simulink library "commsynccomp2"  (Simulink 6.0)
settings: Solver=ode45  SolverMode=SingleTasking  StartTime=0.0  StopTime=10.0  RelTol=1e-3
libraries: commblksprivate x15, dspsigattribs x10, simulink_extras x2, commcontsrc2 x2, dspsrcs4 x1
settings Model: Creator=akansal  LastModifiedBy=cvora  ExtModeAutoUpdateStatusClock=off
settings DataIOCC: SignalLoggingName=logsOut
settings OptimizationCC: BooleanDataType=off
settings DebuggingCC: CheckExecutionContextPreStartOutputMsg=on  CheckExecutionContextRuntimeOutputMsg=on  SolverPrmCheckMsg=none
settings HardwareCC: TargetUnknown=on
settings SFSimCC: SFSimApplyToAllLibs=on  SFSimBuildMode=Incremental

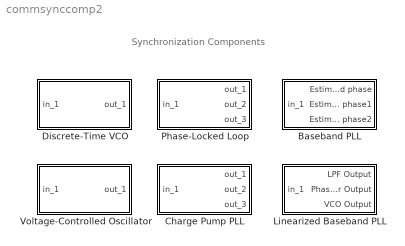
== system commsynccomp2 ==
  note: Synchronization Components
  Baseband PLL : Subsystem  PropExecContextAcrossSSBoundary=on  mask(Baseband PLL){Fn=[3.0002  0  40002], Fd=[1   67.46   2270.9   40002], Kvco=1}
      mask prompts: Fn "Lowpass filter numerator:"; Fd "Lowpass filter denominator:"; Kvco "VCO input sensitivity (Hz/V):"
      mask help: Implement a baseband model of a phase-locked loop. The three outputs are the outputs of the lowpass filter, the phase detector, and the voltage controlled oscillator (VCO). The input must be a sample-based scalar signal.
      mask init:
      | pi2=2*pi;
      mask Help: helpview(commbhelp)
      mask Display:
      | disp('Baseband\nPLL')
      | port_label('output',1,'Filt');
      | port_label('output',2,'PD');
      | port_label('output',3,'VCO');
  Charge Pump PLL : Subsystem  PropExecContextAcrossSSBoundary=on  mask(Charge Pump PLL){Fn=[3.0002  0  40002], Fd=[1   67.46   2270.9   40002], Kvco=1, Fc=100, Ph=0, Ac=1}
      mask prompts: Fn "Lowpass filter numerator:"; Fd "Lowpass filter denominator:"; Kvco "VCO input sensitivity (Hz/V):"; Fc "VCO quiescent frequency (Hz):"; Ph "VCO initial phase (rad):"; Ac "VCO output amplitude (V):"
      mask help: Implement a charge pump phase-locked loop using a digital phase detector. The three outputs are the outputs of the lowpass filter, the phase detector, and the voltage controlled oscillator (VCO). The input must be a sample-based scalar signal.
      mask init:
      | Cu=1;
      mask Help: helpview(commbhelp)
      mask Display:
      | disp('Charge\nPump\nPLL')
      | port_label('output',1,'Filt');
      | port_label('output',2,'PD');
      | port_label('output',3,'VCO');
  Discrete-Time VCO : Subsystem  PropExecContextAcrossSSBoundary=on  mask(Discrete-Time VCO){Ac=1, Fc=10, Kc=1, Ph=0, ts=.01}
      mask prompts: Ac "Output amplitude (V):"; Fc "Quiescent frequency (Hz):"; Kc "Input sensitivity (Hz/V):"; Ph "Initial phase (rad):"; ts "Sample time (s):"
      mask help: Generate a discrete-time output signal whose frequency changes in response to the amplitude variations of the input signal. The input signal must be a scalar.
      mask init:
      | if ((length(Ac)~=1) | (length(Fc)~=1) | (length(Kc)~=1) | (length(Ph)~=1) | (length(ts)~=1))error('Mask parameters must be scalar values.');end;
      | pi2=2*pi;Kc=Kc*pi2*ts(1);Fc=Fc*pi2;
      mask Help: helpview(commbhelp)
      mask Display: disp('Discrete-Time\nVCO')
  Linearized Baseband PLL : Subsystem  PropExecContextAcrossSSBoundary=on  mask(Linearized Baseband PLL){Fn=[3.0002  0  40002], Fd=[1   67.46   2270.9   40002], Kvco=1}
      mask prompts: Fn "Lowpass filter numerator:"; Fd "Lowpass filter denominator:"; Kvco "VCO input sensitivity (Hz/V):"
      mask help: Implement a linearized baseband model of a phase-locked loop. The three outputs are the outputs of the lowpass filter, the phase detector, and the voltage controlled oscillator (VCO). The input must be a sample-based scalar signal.
      mask init:
      | pi2=2*pi;
      mask Help: helpview(commbhelp)
      mask Display:
      | disp('Linearized\nBaseband\nPLL')
      | port_label('output',1,'Filt');
      | port_label('output',2,'PD');
      | port_label('output',3,'VCO');
  Phase-Locked Loop : Subsystem  PropExecContextAcrossSSBoundary=on  mask(Phase-Locked Loop){Fn=[3.0002  0  40002], Fd=[1   67.46   2270.9   40002], Kvco=1, Fc=100, Ph=0, Ac=1}
      mask prompts: Fn "Lowpass filter numerator:"; Fd "Lowpass filter denominator:"; Kvco "VCO input sensitivity (Hz/V):"; Fc "VCO quiescent frequency (Hz):"; Ph "VCO initial phase (rad):"; Ac "VCO output amplitude (V):"
      mask help: Implement a phase-locked loop. The three outputs are: the lowpass filter output, the phase detector output, and the voltage controlled oscillator (VCO) output. The input must be a sample-based scalar signal.
      mask Help: helpview(commbhelp)
      mask Display:
      | disp('PLL')
      | port_label('output',1,'Filt');
      | port_label('output',2,'PD');
      | port_label('output',3,'VCO');
  Voltage-Controlled Oscillator : Subsystem  PropExecContextAcrossSSBoundary=on  mask(Voltage-Controlled Oscillator){Ac=1, Fc=10, Kc=1, Ph=0}
      mask prompts: Ac "Output amplitude (V):"; Fc "Quiescent frequency (Hz):"; Kc "Input sensitivity (Hz/V):"; Ph "Initial phase (rad):"
      mask help: Generate a continuous-time output signal whose frequency changes in response to the amplitude variations of the input signal. The input signal must be a sample-based scalar.
      mask init:
      | if ((length(Ac)~=1) | (length(Fc)~=1) | (length(Ph)~=1) | (length(Kc)~=1) )error('Mask parameters must be scalar values.');end;
      | pi2=2*pi;
      mask Help: helpview(commbhelp)
      mask Display: disp('VCO')

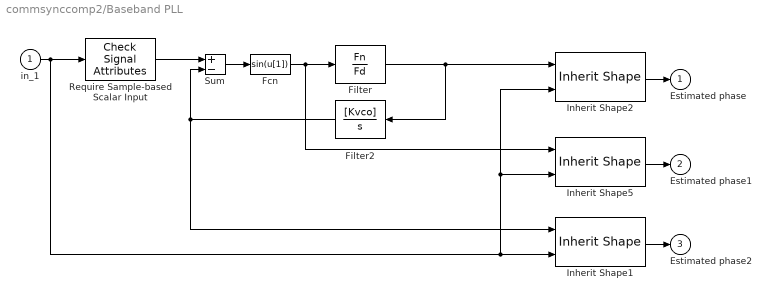
== system commsynccomp2/Baseband PLL ==
  in_1 : Inport  LatchInput=off
  Fcn : Fcn
  Filter : TransferFcn  Numerator=Fn  Denominator=Fd
  Filter2 : TransferFcn  Orientation=left  Numerator=[Kvco]  Denominator=[1 0]
  Inherit Shape1 : commblksprivate/Inherit Shape
  Inherit Shape2 : commblksprivate/Inherit Shape
  Inherit Shape5 : commblksprivate/Inherit Shape
  Require Sample-based Scalar Input : dspsigattribs/Check Signal Attributes  SigAttribCheckMethod=Does not match attributes exactly  Complexity=Ignore  Frame=Sample-based  DimsCheckMethod=Is...  Dimensions=Scalar (1-D or 2-D)  DatatypeCheckMethod=Ignore  DatatypeGeneral=Boolean  DtypeFloatSpecific=Any floating-point  DtypeFixedSpecific=Any fixed-point  DtypeIntSpecific=Any integer  SampleMode=Ignore
  Sum : Sum  Inputs=+-  SaturateOnIntegerOverflow=on  InputSameDT=on
  Estimated phase : Outport  InitialOutput=0
  Estimated phase1 : Outport  Port=2  InitialOutput=0
  Estimated phase2 : Outport  Port=3  InitialOutput=0
  wires:
  Inherit Shape5/1 -> Estimated phase1/1
  Inherit Shape1/1 -> Estimated phase2/1
  Filter2/1 -> Inherit Shape1/1, Sum/2
  Inherit Shape2/1 -> Estimated phase/1
  Require Sample-based Scalar Input/1 -> Sum/1
  Fcn/1 -> Inherit Shape5/1, Filter/1
  Filter/1 -> Inherit Shape2/1, Filter2/1
  Sum/1 -> Fcn/1
  in_1/1 -> Inherit Shape5/2, Inherit Shape2/2, Inherit Shape1/2, Require Sample-based Scalar Input/1

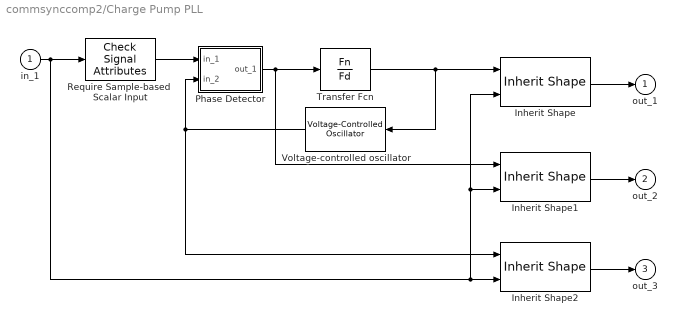
== system commsynccomp2/Charge Pump PLL ==
  in_1 : Inport  LatchInput=off
  Inherit Shape : commblksprivate/Inherit Shape
  Inherit Shape1 : commblksprivate/Inherit Shape
  Inherit Shape2 : commblksprivate/Inherit Shape
  Phase Detector : Subsystem  PropExecContextAcrossSSBoundary=on  mask(Phase Detector){@1=-sqrt(eps), @2=Cu}
      mask prompts: @1 "Cross zero line threshold:"; @2 "Charge pump current:"
      mask help: Phase detector:
      mask init:
      | Thre=@1;Cu=@2;lo=[0 0;0 1;1 0;1 0;0 1;0 1;0 0;0 0;1 0;0 0;1 0;0 0;1 0;0 0;0 0;0 0];
      mask Display: disp('Phase\nDetector')
  Require Sample-based  Scalar Input : dspsigattribs/Check Signal Attributes  SigAttribCheckMethod=Does not match attributes exactly  Complexity=Ignore  Frame=Sample-based  DimsCheckMethod=Is...  Dimensions=Scalar (1-D or 2-D)  DatatypeCheckMethod=Ignore  DatatypeGeneral=Boolean  DtypeFloatSpecific=Any floating-point  DtypeFixedSpecific=Any fixed-point  DtypeIntSpecific=Any integer  SampleMode=Ignore
  Transfer Fcn : TransferFcn  Numerator=Fn  Denominator=Fd
  Voltage-controlled oscillator : commcontsrc2/Voltage-Controlled Oscillator  Orientation=left  Ac=Ac  Fc=Fc  Kc=Kvco  Ph=Ph
  out_1 : Outport  InitialOutput=0
  out_2 : Outport  Port=2  InitialOutput=0
  out_3 : Outport  Port=3  InitialOutput=0
  wires:
  Inherit Shape1/1 -> out_2/1
  Inherit Shape/1 -> out_1/1
  Inherit Shape2/1 -> out_3/1
  Require Sample-based  Scalar Input/1 -> Phase Detector/1(in_1)
  Phase Detector/1(out_1) -> Inherit Shape1/1, Transfer Fcn/1
  Voltage-controlled oscillator/1 -> Inherit Shape2/1, Phase Detector/2(in_2)
  in_1/1 -> Inherit Shape/2, Inherit Shape1/2, Inherit Shape2/2, Require Sample-based  Scalar Input/1
  Transfer Fcn/1 -> Inherit Shape/1, Voltage-controlled oscillator/1

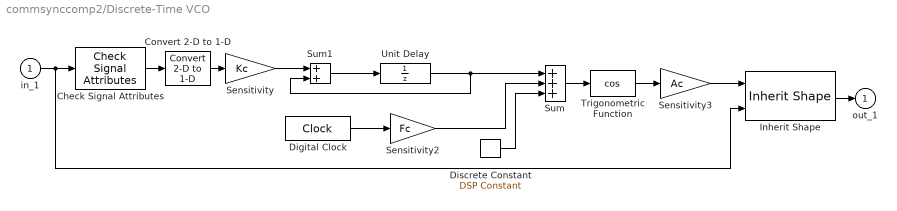
== system commsynccomp2/Discrete-Time VCO ==
  in_1 : Inport  LatchInput=off
  Check Signal Attributes : dspsigattribs/Check Signal Attributes  SigAttribCheckMethod=Does not match attributes exactly  Complexity=Ignore  Frame=Ignore  DimsCheckMethod=Is...  Dimensions=Scalar (1-D or 2-D)  DatatypeCheckMethod=Ignore  DatatypeGeneral=Boolean  DtypeFloatSpecific=Any floating-point  DtypeFixedSpecific=Any fixed-point  DtypeIntSpecific=Any integer  SampleMode=Ignore
  Convert 2-D to 1-D : dspsigattribs/Convert 2-D to 1-D
  Digital Clock : DigitalClock  SampleTime=ts
  Discrete Constant : dspsrcs4/DSP Constant  Value=Ph  SampleMode=Discrete  discreteOutput=Sample-based (interpret vectors as 1-D)  continuousOutput=Sample-based  sampTime=ts  framePeriod=ts  dataType=Inherit from 'Constant value'  wordLen=16  udDataType=sfix(16)  fracBitsMode=Best precision  numFracBits=15  InterpretAs1D=on  Ts=ts  FramebasedOutput=off
  Inherit Shape : commblksprivate/Inherit Shape
  Sensitivity : Gain  Gain=Kc  SaturateOnIntegerOverflow=on
  Sensitivity2 : Gain  Gain=Fc  SaturateOnIntegerOverflow=on
  Sensitivity3 : Gain  Gain=Ac  SaturateOnIntegerOverflow=on
  Sum : Sum  Inputs=+++  SaturateOnIntegerOverflow=on  InputSameDT=on
  Sum1 : Sum  SaturateOnIntegerOverflow=on  InputSameDT=on
  Trigonometric Function : Trigonometry  Operator=cos
  Unit Delay : UnitDelay  SampleTime=ts
  out_1 : Outport  InitialOutput=0
  wires:
  in_1/1 -> Inherit Shape/2, Check Signal Attributes/1
  Sensitivity/1 -> Sum1/1
  Sum1/1 -> Unit Delay/1
  Sum/1 -> Trigonometric Function/1
  Digital Clock/1 -> Sensitivity2/1
  Sensitivity2/1 -> Sum/2
  Unit Delay/1 -> Sum/1, Sum1/2
  Discrete Constant/1 -> Sum/3
  Trigonometric Function/1 -> Sensitivity3/1
  Convert 2-D to 1-D/1 -> Sensitivity/1
  Sensitivity3/1 -> Inherit Shape/1
  Inherit Shape/1 -> out_1/1
  Check Signal Attributes/1 -> Convert 2-D to 1-D/1

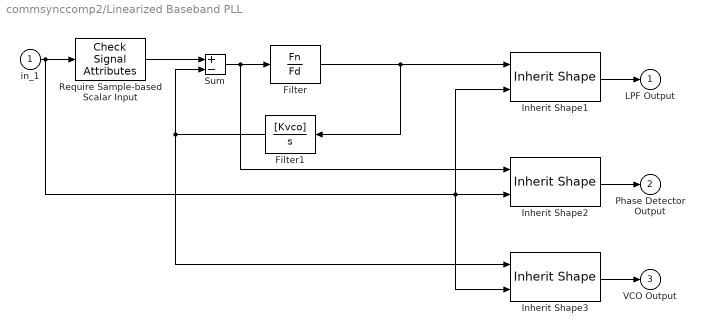
== system commsynccomp2/Linearized Baseband PLL ==
  in_1 : Inport  LatchInput=off
  Filter : TransferFcn  Numerator=Fn  Denominator=Fd
  Filter1 : TransferFcn  Orientation=left  Numerator=[Kvco]  Denominator=[1 0]
  Inherit Shape1 : commblksprivate/Inherit Shape
  Inherit Shape2 : commblksprivate/Inherit Shape
  Inherit Shape3 : commblksprivate/Inherit Shape
  Require Sample-based Scalar Input : dspsigattribs/Check Signal Attributes  SigAttribCheckMethod=Does not match attributes exactly  Complexity=Ignore  Frame=Sample-based  DimsCheckMethod=Is...  Dimensions=Scalar (1-D or 2-D)  DatatypeCheckMethod=Ignore  DatatypeGeneral=Boolean  DtypeFloatSpecific=Any floating-point  DtypeFixedSpecific=Any fixed-point  DtypeIntSpecific=Any integer  SampleMode=Ignore
  Sum : Sum  Inputs=+-  SaturateOnIntegerOverflow=on  InputSameDT=on
  LPF Output : Outport  InitialOutput=0
  Phase Detector Output : Outport  Port=2  InitialOutput=0
  VCO Output : Outport  Port=3  InitialOutput=0
  wires:
  Inherit Shape2/1 -> Phase Detector Output/1
  Inherit Shape3/1 -> VCO Output/1
  Inherit Shape1/1 -> LPF Output/1
  Require Sample-based Scalar Input/1 -> Sum/1
  Sum/1 -> Inherit Shape2/1, Filter/1
  Filter/1 -> Inherit Shape1/1, Filter1/1
  Filter1/1 -> Inherit Shape3/1, Sum/2
  in_1/1 -> Inherit Shape2/2, Inherit Shape3/2, Inherit Shape1/2, Require Sample-based Scalar Input/1

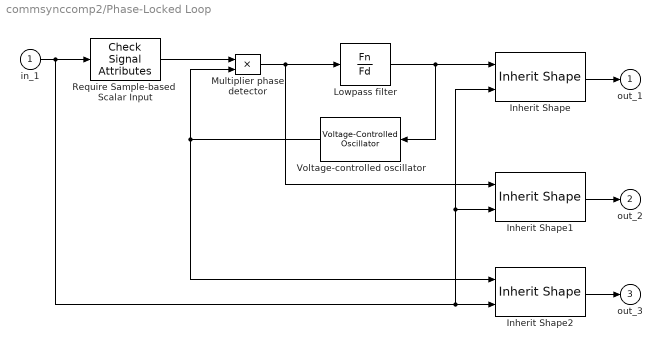
== system commsynccomp2/Phase-Locked Loop ==
  in_1 : Inport  LatchInput=off
  Inherit Shape : commblksprivate/Inherit Shape
  Inherit Shape1 : commblksprivate/Inherit Shape
  Inherit Shape2 : commblksprivate/Inherit Shape
  Lowpass filter : TransferFcn  Numerator=Fn  Denominator=Fd
  Multiplier phase detector : Product  SaturateOnIntegerOverflow=on  InputSameDT=on
  Require Sample-based  Scalar Input : dspsigattribs/Check Signal Attributes  SigAttribCheckMethod=Does not match attributes exactly  Complexity=Ignore  Frame=Sample-based  DimsCheckMethod=Is...  Dimensions=Scalar (1-D or 2-D)  DatatypeCheckMethod=Ignore  DatatypeGeneral=Boolean  DtypeFloatSpecific=Any floating-point  DtypeFixedSpecific=Any fixed-point  DtypeIntSpecific=Any integer  SampleMode=Ignore
  Voltage-controlled oscillator : commcontsrc2/Voltage-Controlled Oscillator  Orientation=left  Ac=Ac  Fc=Fc  Kc=Kvco  Ph=Ph
  out_1 : Outport  InitialOutput=0
  out_2 : Outport  Port=2  InitialOutput=0
  out_3 : Outport  Port=3  InitialOutput=0
  wires:
  Inherit Shape1/1 -> out_2/1
  Inherit Shape2/1 -> out_3/1
  Inherit Shape/1 -> out_1/1
  Require Sample-based  Scalar Input/1 -> Multiplier phase detector/1
  Voltage-controlled oscillator/1 -> Inherit Shape2/1, Multiplier phase detector/2
  Multiplier phase detector/1 -> Inherit Shape1/1, Lowpass filter/1
  in_1/1 -> Inherit Shape/2, Inherit Shape1/2, Inherit Shape2/2, Require Sample-based  Scalar Input/1
  Lowpass filter/1 -> Inherit Shape/1, Voltage-controlled oscillator/1

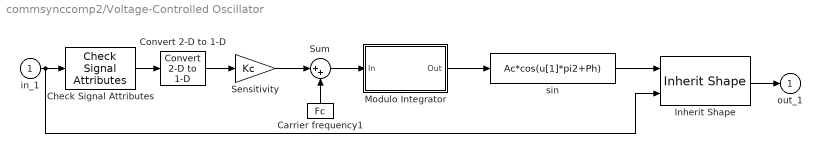
== system commsynccomp2/Voltage-Controlled Oscillator ==
  in_1 : Inport  LatchInput=off
  Carrier frequency1 : Constant  Orientation=up  Value=Fc
  Check Signal Attributes : dspsigattribs/Check Signal Attributes  SigAttribCheckMethod=Does not match attributes exactly  Complexity=Ignore  Frame=Sample-based  DimsCheckMethod=Is...  Dimensions=Scalar (1-D or 2-D)  DatatypeCheckMethod=Ignore  DatatypeGeneral=Boolean  DtypeFloatSpecific=Any floating-point  DtypeFixedSpecific=Any fixed-point  DtypeIntSpecific=Any integer  SampleMode=Ignore
  Convert 2-D to 1-D : dspsigattribs/Convert 2-D to 1-D
  Inherit Shape : commblksprivate/Inherit Shape
  Modulo Integrator : Subsystem  PropExecContextAcrossSSBoundary=on  mask(Modulo Integrator){modu=1, init=0}
      mask prompts: modu "Absolute value bound:"; init "Initial condition:"
      mask help:
      | Integrate the input signal in continuous time and then uses the Absolute value bound parameter, K, to produce output strictly between -K and K. The block uses the rem function in MATLAB.
      |
      | The input must be sample-based.
      mask init:
      | [modu, init]=commblkmodint(gcb);
      mask Help: helpview(commbhelp)
      mask Display: disp('Modulo\nIntegrator')
  Sensitivity : Gain  Gain=Kc  SaturateOnIntegerOverflow=on
  Sum : Sum  Inputs=|++  SaturateOnIntegerOverflow=on  InputSameDT=on
  sin : Fcn  Expr=Ac*cos(u[1]*pi2+Ph)
  out_1 : Outport  InitialOutput=0
  wires:
  Sum/1 -> Modulo Integrator/1(In)
  Modulo Integrator/1(Out) -> sin/1
  Carrier frequency1/1 -> Sum/2
  Sensitivity/1 -> Sum/1
  in_1/1 -> Inherit Shape/2, Check Signal Attributes/1
  Convert 2-D to 1-D/1 -> Sensitivity/1
  sin/1 -> Inherit Shape/1
  Inherit Shape/1 -> out_1/1
  Check Signal Attributes/1 -> Convert 2-D to 1-D/1

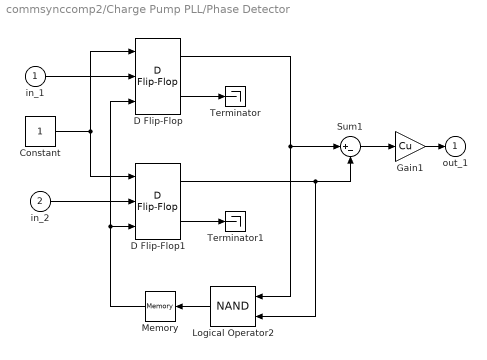
== system commsynccomp2/Charge Pump PLL/Phase Detector ==
  in_1 : Inport  LatchInput=off
  in_2 : Inport  Port=2  LatchInput=off
  Constant : Constant  OutDataTypeMode=boolean
  D Flip-Flop : simulink_extras/Flip Flops/D Flip-Flop
  D Flip-Flop1 : simulink_extras/Flip Flops/D Flip-Flop
  Gain1 : Gain  Gain=Cu  SaturateOnIntegerOverflow=on
  Logical Operator2 : Logic  Orientation=left  Operator=NAND
  Memory : Memory  Orientation=left
  Sum1 : Sum  Inputs=|+-  OutDataTypeMode=double  SaturateOnIntegerOverflow=on  InputSameDT=on
  Terminator : Terminator
  Terminator1 : Terminator
  out_1 : Outport  InitialOutput=0
  wires:
  Memory/1 -> D Flip-Flop/3, D Flip-Flop1/3
  Logical Operator2/1 -> Memory/1
  D Flip-Flop1/1 -> Logical Operator2/2, Sum1/2
  Gain1/1 -> out_1/1
  D Flip-Flop/1 -> Logical Operator2/1, Sum1/1
  D Flip-Flop1/2 -> Terminator1/1
  D Flip-Flop/2 -> Terminator/1
  Constant/1 -> D Flip-Flop/1, D Flip-Flop1/1
  in_2/1 -> D Flip-Flop1/2
  in_1/1 -> D Flip-Flop/2
  Sum1/1 -> Gain1/1

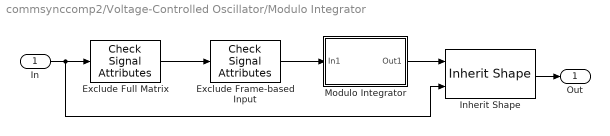
== system commsynccomp2/Voltage-Controlled Oscillator/Modulo Integrator ==
  In : Inport  LatchInput=off
  "Exclude Frame-based Input " : dspsigattribs/Check Signal Attributes  SigAttribCheckMethod=Matches attributes exactly  Complexity=Ignore  Frame=Frame-based  DimsCheckMethod=Ignore  Dimensions=Scalar (1-D or 2-D)  DatatypeCheckMethod=Ignore  DatatypeGeneral=Boolean  DtypeFloatSpecific=Any floating-point  DtypeFixedSpecific=Any fixed-point  DtypeIntSpecific=Any integer  SampleMode=Ignore
  Exclude Full Matrix : dspsigattribs/Check Signal Attributes  SigAttribCheckMethod=Matches attributes exactly  Complexity=Ignore  Frame=Ignore  DimsCheckMethod=Is...  Dimensions=Full matrix (2-D)  DatatypeCheckMethod=Ignore  DatatypeGeneral=Boolean  DtypeFloatSpecific=Any floating-point  DtypeFixedSpecific=Any fixed-point  DtypeIntSpecific=Any integer  SampleMode=Ignore
  Inherit Shape : commblksprivate/Inherit Shape
  Modulo Integrator : Subsystem  PropExecContextAcrossSSBoundary=on
  Out : Outport
  wires:
  Exclude Full Matrix/1 -> "Exclude Frame-based Input "/1
  "Exclude Frame-based Input "/1 -> Modulo Integrator/1(In1)
  In/1 -> Exclude Full Matrix/1, Inherit Shape/2
  Modulo Integrator/1(Out1) -> Inherit Shape/1
  Inherit Shape/1 -> Out/1

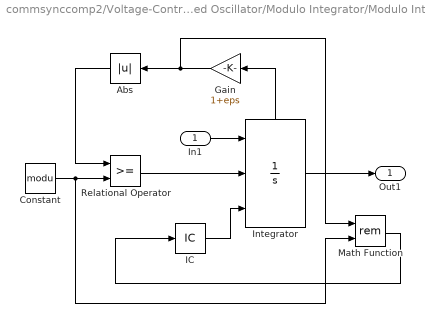
== system commsynccomp2/Voltage-Controlled Oscillator/Modulo Integrator/Modulo Integrator ==
  In1 : Inport  LatchInput=off
  Abs : Abs  Orientation=left  SaturateOnIntegerOverflow=on
  Constant : Constant  Value=modu
  Gain : Gain  Orientation=left  Gain=1+eps  SaturateOnIntegerOverflow=on
  IC : InitialCondition  Value=init
  Integrator : Integrator  ExternalReset=rising  InitialConditionSource=external  UpperSaturationLimit=1  LowerSaturationLimit=0  ShowStatePort=on
  Math Function : Math  Operator=rem  SaturateOnIntegerOverflow=on
  Relational Operator : RelationalOperator  InputSameDT=on
  Out1 : Outport
  wires:
  IC/1 -> Integrator/3
  In1/1 -> Integrator/1
  Integrator/1 -> Out1/1
  Math Function/1 -> IC/1
  Abs/1 -> Relational Operator/1
  Relational Operator/1 -> Integrator/2
  Constant/1 -> Math Function/2, Relational Operator/2
  Integrator/State -> Gain/1
  Gain/1 -> Abs/1, Math Function/1
